simulink model "Mohinhmoi"  (R2018a)
settings: Solver=ode5  StartTime=0.0  StopTime=1000  FixedStep=0.05  RelTol=1e-3
settings Model: PacingRate=100  Creator=Hungs  LastModifiedBy=Hungs

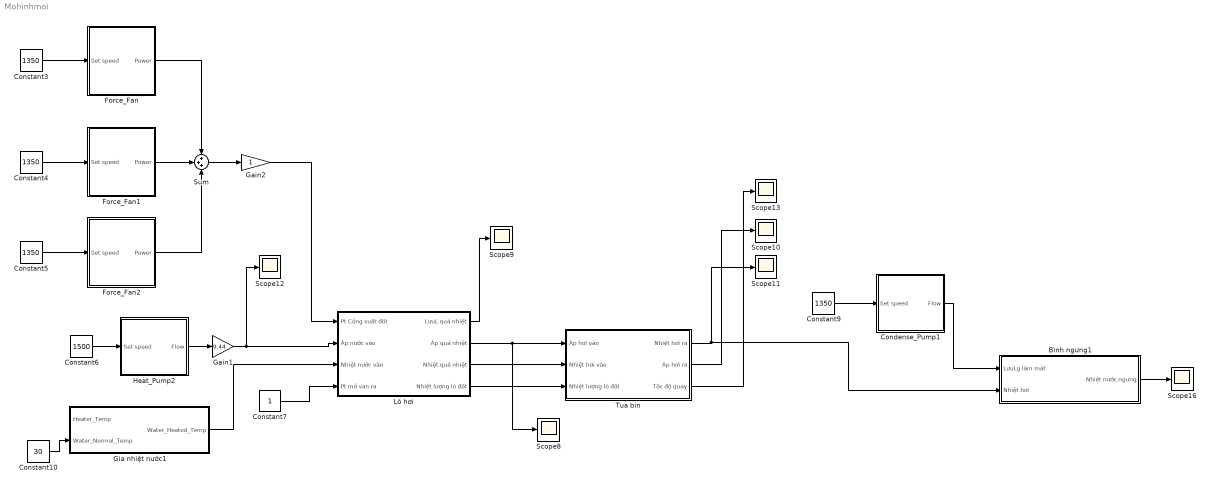
== system Mohinhmoi ==
  Bình ngưng1 : Subsystem
  Condense_Pump1 : Subsystem
      mask Display: image('C:\Program Files\MATLAB\ThermalElectricity\Maskicon\Pump.png');
  Constant10 : Constant  Value=30
  Constant{3..5,9} (4 alike) : Constant  Value=1350
  Constant6 : Constant  Value=1500
  Constant7 : Constant
  Force_Fan : Subsystem
      mask Display: image('C:\Program Files\MATLAB\ThermalElectricity\Maskicon\Fan.png');
  Force_Fan1 : Subsystem
      mask Display: image('C:\Program Files\MATLAB\ThermalElectricity\Maskicon\Fan.png');
  Force_Fan2 : Subsystem
      mask Display: image('C:\Program Files\MATLAB\ThermalElectricity\Maskicon\Fan.png');
  Gain1 : Gain  Gain=9.44
  Gain2 : Gain
  Gia nhiệt nước1 : Subsystem
  Heat_Pump2 : Subsystem
  Lò hơi : Subsystem
  Scope{8..13,16} (7 alike) : Scope
  Sum : Sum  Inputs=+++
  Tua bin : Subsystem
  wires:
  Gain2/1 -> Lò hơi/1(Pt Công suất đốt)
  Heat_Pump2/1(Flow) -> Gain1/1
  Constant6/1 -> Heat_Pump2/1(Set speed)
  Gain1/1 -> Scope12/1, Lò hơi/2(Áp nước vào)
  Constant7/1 -> Lò hơi/4(Pt mở van ra)
  Lò hơi/1(LưuL quá nhiệt) -> Scope9/1
  Lò hơi/2(Áp quá nhiệt) -> Scope8/1, Tua bin/1(Áp hơi vào)
  Gia nhiệt nước1/1(Water_Heated_Temp) -> Lò hơi/3(Nhiệt nước vào)
  Lò hơi/3(Nhiệt quá nhiệt) -> Tua bin/2(Nhiệt hơi vào)
  Lò hơi/4(Nhiệt lượng lò đốt) -> Tua bin/3(Nhiệt lượng lò đốt)
  Tua bin/2(Áp hơi ra) -> Scope10/1
  Tua bin/3(Tốc độ quay) -> Scope13/1
  Bình ngưng1/1(Nhiệt nước ngưng) -> Scope16/1
  Condense_Pump1/1(Flow) -> Bình ngưng1/1(LưuLg làm mát)
  Tua bin/1(Nhiệt hơi ra) -> Bình ngưng1/2(Nhiệt hơi), Scope11/1
  Constant9/1 -> Condense_Pump1/1(Set speed)
  Constant10/1 -> Gia nhiệt nước1/2(Water_Normal_Temp)
  Force_Fan/1(Power) -> Sum/1
  Constant4/1 -> Force_Fan1/1(Set speed)
  Sum/1 -> Gain2/1
  Constant5/1 -> Force_Fan2/1(Set speed)
  Force_Fan2/1(Power) -> Sum/3
  Constant3/1 -> Force_Fan/1(Set speed)
  Force_Fan1/1(Power) -> Sum/2

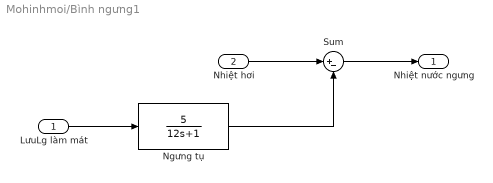
== system Mohinhmoi/Bình ngưng1 ==
  LưuLg làm mát : Inport
  Nhiệt hơi : Inport  Port=2
  Ngưng tụ : TransferFcn  Numerator=[5]  Denominator=[12 1]
  Sum : Sum  Inputs=|+-
  Nhiệt nước ngưng : Outport
  wires:
  Sum/1 -> Nhiệt nước ngưng/1
  Ngưng tụ/1 -> Sum/2
  Nhiệt hơi/1 -> Sum/1
  LưuLg làm mát/1 -> Ngưng tụ/1

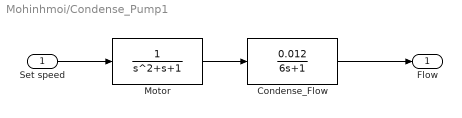
== system Mohinhmoi/Condense_Pump1 ==
  Set speed : Inport
  Condense_Flow : TransferFcn  Numerator=[0.012]  Denominator=[6 1]
  Motor : TransferFcn  Denominator=[1 1 1]
  Flow : Outport
  wires:
  Motor/1 -> Condense_Flow/1
  Set speed/1 -> Motor/1
  Condense_Flow/1 -> Flow/1

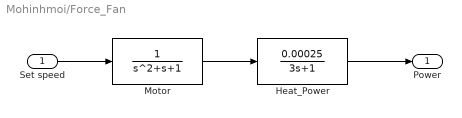
== system Mohinhmoi/Force_Fan ==
  Set speed : Inport
  Heat_Power : TransferFcn  Numerator=[0.00025]  Denominator=[3 1]
  Motor : TransferFcn  Denominator=[1 1 1]
  Power : Outport
  wires:
  Motor/1 -> Heat_Power/1
  Set speed/1 -> Motor/1
  Heat_Power/1 -> Power/1

== system Mohinhmoi/Force_Fan1 ==
  Set speed : Inport
  Heat_Power : TransferFcn  Numerator=[0.00025]  Denominator=[3 1]
  Motor : TransferFcn  Denominator=[1 1 1]
  Power : Outport
  wires:
  Heat_Power/1 -> Power/1
  Set speed/1 -> Motor/1
  Motor/1 -> Heat_Power/1

== system Mohinhmoi/Force_Fan2 ==
  Set speed : Inport
  Heat_Power : TransferFcn  Numerator=[0.00025]  Denominator=[3 1]
  Motor : TransferFcn  Denominator=[1 1 1]
  Power : Outport
  wires:
  Motor/1 -> Heat_Power/1
  Set speed/1 -> Motor/1
  Heat_Power/1 -> Power/1

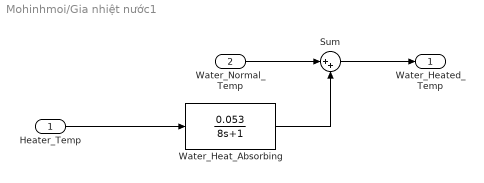
== system Mohinhmoi/Gia nhiệt nước1 ==
  Heater_Temp : Inport
  Water_Normal_Temp : Inport  Port=2
  Sum : Sum  Inputs=|++
  Water_Heat_Absorbing : TransferFcn  Numerator=[0.053]  Denominator=[8 1]
  Water_Heated_Temp : Outport
  wires:
  Heater_Temp/1 -> Water_Heat_Absorbing/1
  Water_Normal_Temp/1 -> Sum/1
  Water_Heat_Absorbing/1 -> Sum/2
  Sum/1 -> Water_Heated_Temp/1

== system Mohinhmoi/Heat_Pump2 ==
  Set speed : Inport
  Heat_Flow : TransferFcn  Numerator=[0.0178]  Denominator=[10 1]
  Motor : TransferFcn  Denominator=[1 1 1]
  Flow : Outport
  wires:
  Motor/1 -> Heat_Flow/1
  Set speed/1 -> Motor/1
  Heat_Flow/1 -> Flow/1

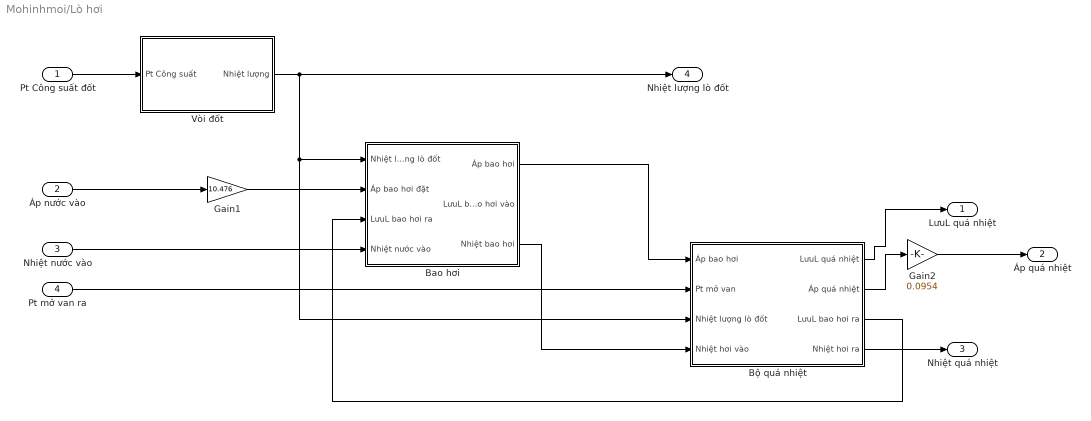
== system Mohinhmoi/Lò hơi ==
  Pt Công suất đốt : Inport
  Áp nước vào : Inport  Port=2
  Nhiệt nước vào : Inport  Port=3
  Pt mở van ra : Inport  Port=4
  Bao hơi : Subsystem  mask{Cm=0.3, Kw=0.04, Kt=0.000025, Kh=-300, Cd=150}
      mask prompts: Cm "Hệ số hấp thụ nhiệt ống sinh hơi"; Kw "Hệ số truyền nhiệt ống sinh hơi"; Kt "Tỉ lệ áp suất - nhiệt độ trong ống sinh hơi"; Kh "Hệ số biến thiên entanpi theo áp suất bao hơi"; Cd "Thời hằng bao hơi"
  Bộ quá nhiệt : Subsystem  mask{K=44, Cs=20}
      mask prompts: K "Hệ số tụt áp"; Cs "Thời hằng bộ quá nhiệt"
  Gain1 : Gain  Gain=10.476
  Gain2 : Gain  Gain=0.0954
  Vòi đốt : Subsystem  mask{Tf=100, Td=20}
      mask prompts: Tf "Thời hằng vòi đốt"; Td "Thời gian trễ vòi đốt"
  LưuL quá nhiệt : Outport
  Áp quá nhiệt : Outport  Port=2
  Nhiệt quá nhiệt : Outport  Port=3
  Nhiệt lượng lò đốt : Outport  Port=4
  wires:
  Bộ quá nhiệt/1(LưuL quá nhiệt) -> LưuL quá nhiệt/1
  Bộ quá nhiệt/2(Áp quá nhiệt) -> Gain2/1
  Bao hơi/1(Áp bao hơi) -> Bộ quá nhiệt/1(Áp bao hơi)
  Vòi đốt/1(Nhiệt lượng) -> Nhiệt lượng lò đốt/1, Bộ quá nhiệt/3(Nhiệt lượng lò đốt), Bao hơi/1(Nhiệt lượng lò đốt)
  Bộ quá nhiệt/3(LưuL bao hơi ra) -> Bao hơi/3(LưuL bao hơi ra)
  Áp nước vào/1 -> Gain1/1
  Pt mở van ra/1 -> Bộ quá nhiệt/2(Pt mở van)
  Pt Công suất đốt/1 -> Vòi đốt/1(Pt Công suất)
  Gain1/1 -> Bao hơi/2(Áp bao hơi đặt)
  Gain2/1 -> Áp quá nhiệt/1
  Nhiệt nước vào/1 -> Bao hơi/4(Nhiệt nước vào)
  Bao hơi/3(Nhiệt bao hơi) -> Bộ quá nhiệt/4(Nhiệt hơi vào)
  Bộ quá nhiệt/4(Nhiệt hơi ra) -> Nhiệt quá nhiệt/1

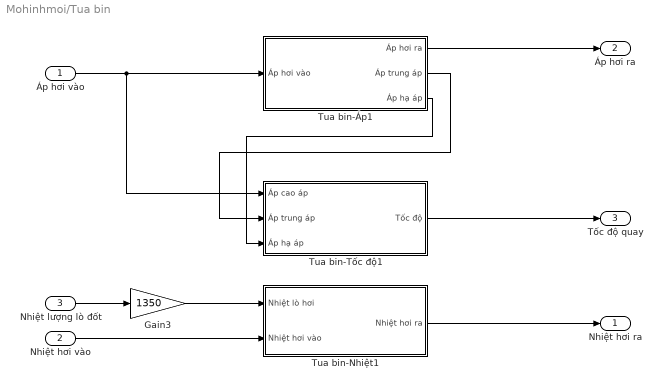
== system Mohinhmoi/Tua bin ==
  Áp hơi vào : Inport
  Nhiệt hơi vào : Inport  Port=2
  Nhiệt lượng lò đốt : Inport  Port=3
  Gain3 : Gain  Gain=1350
  Tua bin-Nhiệt1 : Subsystem
  Tua bin-Tốc độ1 : Subsystem
  Tua bin-Áp1 : Subsystem
  Nhiệt hơi ra : Outport
  Áp hơi ra : Outport  Port=2
  Tốc độ quay : Outport  Port=3
  wires:
  Tua bin-Áp1/3(Áp hạ áp) -> Tua bin-Tốc độ1/3(Áp hạ áp)
  Tua bin-Áp1/2(Áp trung áp) -> Tua bin-Tốc độ1/2(Áp trung áp)
  Áp hơi vào/1 -> Tua bin-Tốc độ1/1(Áp cao áp), Tua bin-Áp1/1(Áp hơi vào)
  Nhiệt lượng lò đốt/1 -> Gain3/1
  Nhiệt hơi vào/1 -> Tua bin-Nhiệt1/2(Nhiệt hơi vào)
  Tua bin-Nhiệt1/1(Nhiệt hơi ra) -> Nhiệt hơi ra/1
  Tua bin-Áp1/1(Áp hơi ra) -> Áp hơi ra/1
  Tua bin-Tốc độ1/1(Tốc độ) -> Tốc độ quay/1
  Gain3/1 -> Tua bin-Nhiệt1/1(Nhiệt lò hơi)

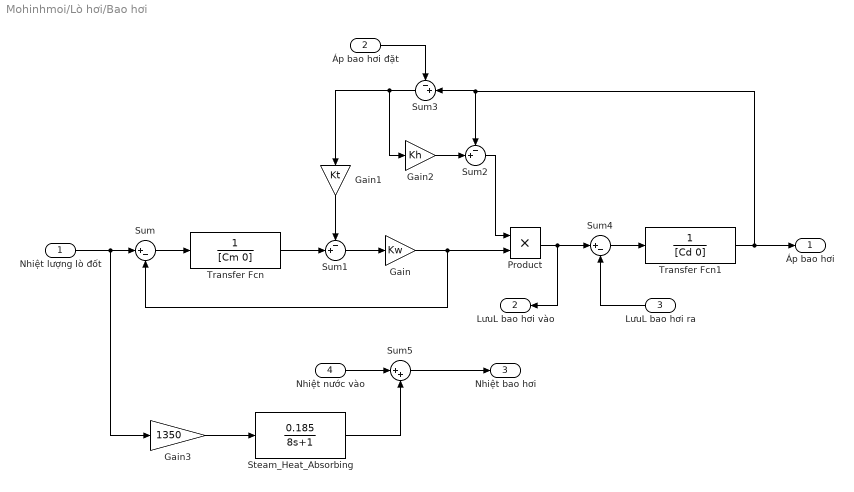
== system Mohinhmoi/Lò hơi/Bao hơi ==
  Nhiệt lượng lò đốt : Inport
  Áp bao hơi đặt : Inport  Port=2
  LưuL bao hơi ra : Inport  Port=3
  Nhiệt nước vào : Inport  Port=4
  Gain : Gain  Gain=Kw
  Gain1 : Gain  Gain=Kt
  Gain2 : Gain  Gain=Kh
  Gain3 : Gain  Gain=1350
  Product : Product
  Steam_Heat_Absorbing : TransferFcn  Numerator=[0.185]  Denominator=[8 1]
  Sum : Sum  Inputs=|+-
  Sum1 : Sum  Inputs=-+|
  Sum2 : Sum  Inputs=-+|
  Sum3 : Sum  Inputs=-+|
  Sum4 : Sum  Inputs=|+-
  Sum5 : Sum  Inputs=|++
  Transfer Fcn : TransferFcn  Denominator=[Cm 0]
  Transfer Fcn1 : TransferFcn  Denominator=[Cd 0]
  Áp bao hơi : Outport
  LưuL bao hơi vào : Outport  Port=2
  Nhiệt bao hơi : Outport  Port=3
  wires:
  Transfer Fcn/1 -> Sum1/2
  Sum1/1 -> Gain/1
  Gain/1 -> Product/2, Sum/2
  Sum/1 -> Transfer Fcn/1
  Gain1/1 -> Sum1/1
  Transfer Fcn1/1 -> Áp bao hơi/1, Sum2/1, Sum3/2
  Sum2/1 -> Product/1
  Gain2/1 -> Sum2/2
  Sum3/1 -> Gain1/1, Gain2/1
  Áp bao hơi đặt/1 -> Sum3/1
  Product/1 -> Sum4/1, LưuL bao hơi vào/1
  LưuL bao hơi ra/1 -> Sum4/2
  Sum4/1 -> Transfer Fcn1/1
  Nhiệt lượng lò đốt/1 -> Sum/1, Gain3/1
  Steam_Heat_Absorbing/1 -> Sum5/2
  Nhiệt nước vào/1 -> Sum5/1
  Sum5/1 -> Nhiệt bao hơi/1
  Gain3/1 -> Steam_Heat_Absorbing/1

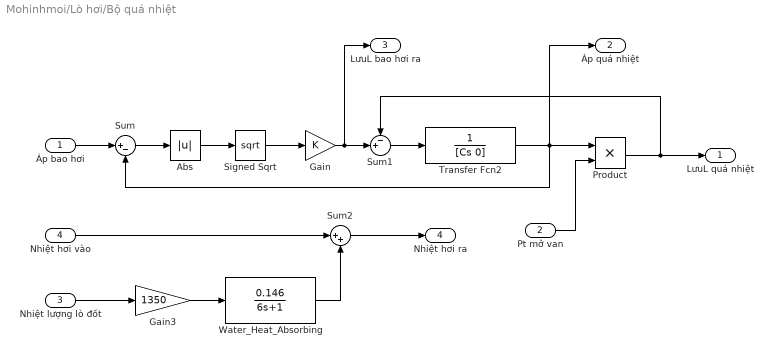
== system Mohinhmoi/Lò hơi/Bộ quá nhiệt ==
  Áp bao hơi : Inport
  Pt mở van : Inport  Port=2
  Nhiệt lượng lò đốt : Inport  Port=3
  Nhiệt hơi vào : Inport  Port=4
  Abs : Abs
  Gain : Gain  Gain=K
  Gain3 : Gain  Gain=1350
  Product : Product
  Signed Sqrt : Sqrt  SaturateOnIntegerOverflow=on
  Sum : Sum  Inputs=|+-
  Sum1 : Sum  Inputs=-+|
  Sum2 : Sum  Inputs=|++
  Transfer Fcn2 : TransferFcn  Denominator=[Cs 0]
  Water_Heat_Absorbing : TransferFcn  Numerator=[0.146]  Denominator=[6 1]
  LưuL quá nhiệt : Outport
  Áp quá nhiệt : Outport  Port=2
  LưuL bao hơi ra : Outport  Port=3
  Nhiệt hơi ra : Outport  Port=4
  wires:
  Transfer Fcn2/1 -> Áp quá nhiệt/1, Sum/2, Product/1
  Áp bao hơi/1 -> Sum/1
  Sum/1 -> Abs/1
  Abs/1 -> Signed Sqrt/1
  Signed Sqrt/1 -> Gain/1
  Pt mở van/1 -> Product/2
  Gain/1 -> LưuL bao hơi ra/1, Sum1/2
  Sum1/1 -> Transfer Fcn2/1
  Product/1 -> LưuL quá nhiệt/1, Sum1/1
  Nhiệt hơi vào/1 -> Sum2/1
  Water_Heat_Absorbing/1 -> Sum2/2
  Nhiệt lượng lò đốt/1 -> Gain3/1
  Sum2/1 -> Nhiệt hơi ra/1
  Gain3/1 -> Water_Heat_Absorbing/1

== system Mohinhmoi/Lò hơi/Vòi đốt ==
  Pt Công suất : Inport
  Furnace : TransferFcn  Denominator=[Tf 1]
  Transport Delay : TransportDelay  DelayTime=Td
  Nhiệt lượng : Outport
  wires:
  Pt Công suất/1 -> Furnace/1
  Furnace/1 -> Transport Delay/1
  Transport Delay/1 -> Nhiệt lượng/1

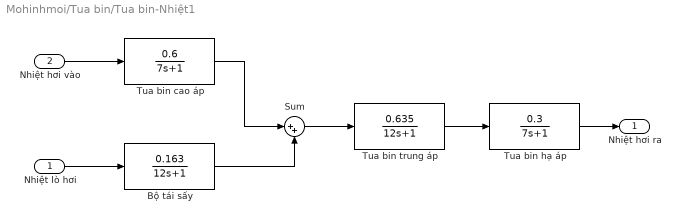
== system Mohinhmoi/Tua bin/Tua bin-Nhiệt1 ==
  Nhiệt lò hơi : Inport
  Nhiệt hơi vào : Inport  Port=2
  Bộ tái sấy : TransferFcn  Numerator=[0.163]  Denominator=[12 1]
  Sum : Sum  Inputs=|++
  Tua bin cao áp : TransferFcn  Numerator=[0.6]  Denominator=[7 1]
  Tua bin hạ áp : TransferFcn  Numerator=[0.3]  Denominator=[7 1]
  Tua bin trung áp : TransferFcn  Numerator=[0.635]  Denominator=[12 1]
  Nhiệt hơi ra : Outport
  wires:
  Tua bin hạ áp/1 -> Nhiệt hơi ra/1
  Tua bin trung áp/1 -> Tua bin hạ áp/1
  Sum/1 -> Tua bin trung áp/1
  Tua bin cao áp/1 -> Sum/1
  Nhiệt hơi vào/1 -> Tua bin cao áp/1
  Bộ tái sấy/1 -> Sum/2
  Nhiệt lò hơi/1 -> Bộ tái sấy/1

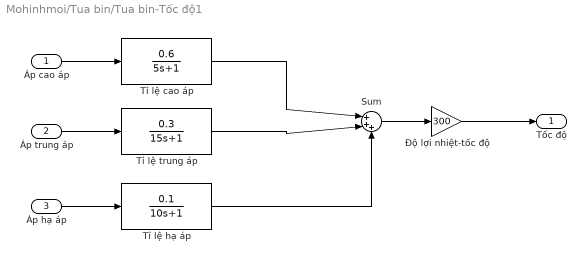
== system Mohinhmoi/Tua bin/Tua bin-Tốc độ1 ==
  Áp cao áp : Inport
  Áp trung áp : Inport  Port=2
  Áp hạ áp : Inport  Port=3
  Sum : Sum  Inputs=|+++
  Tỉ lệ cao áp : TransferFcn  Numerator=[0.6]  Denominator=[5 1]
  Tỉ lệ hạ áp : TransferFcn  Numerator=[0.1]  Denominator=[10 1]
  Tỉ lệ trung áp : TransferFcn  Numerator=[0.3]  Denominator=[15 1]
  Độ lợi nhiệt-tốc độ : Gain  Gain=300
  Tốc độ : Outport
  wires:
  Áp cao áp/1 -> Tỉ lệ cao áp/1
  Tỉ lệ cao áp/1 -> Sum/1
  Sum/1 -> Độ lợi nhiệt-tốc độ/1
  Áp trung áp/1 -> Tỉ lệ trung áp/1
  Áp hạ áp/1 -> Tỉ lệ hạ áp/1
  Tỉ lệ trung áp/1 -> Sum/2
  Tỉ lệ hạ áp/1 -> Sum/3
  Độ lợi nhiệt-tốc độ/1 -> Tốc độ/1

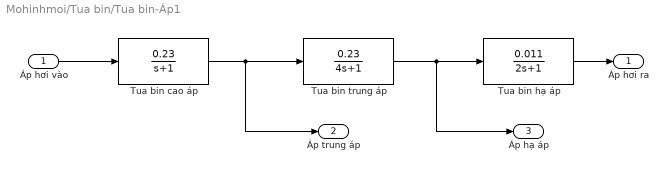
== system Mohinhmoi/Tua bin/Tua bin-Áp1 ==
  Áp hơi vào : Inport
  Tua bin cao áp : TransferFcn  Numerator=[0.23]  Denominator=[1 1]
  Tua bin hạ áp : TransferFcn  Numerator=[0.011]  Denominator=[2 1]
  Tua bin trung áp : TransferFcn  Numerator=[0.23]  Denominator=[4 1]
  Áp hơi ra : Outport
  Áp trung áp : Outport  Port=2
  Áp hạ áp : Outport  Port=3
  wires:
  Tua bin hạ áp/1 -> Áp hơi ra/1
  Tua bin trung áp/1 -> Áp hạ áp/1, Tua bin hạ áp/1
  Tua bin cao áp/1 -> Áp trung áp/1, Tua bin trung áp/1
  Áp hơi vào/1 -> Tua bin cao áp/1
